simulink model "gm_gmStateSpaceHDL_HalfWaveRectifier_HDL"  (R2020b)
settings: Solver=FixedStepDiscrete  StartTime=0.0  StopTime=5*tin  RelTol=1e-3  AbsTol=1e-3
InitFcn:
  | ts = 1e-6; % local solver sample time
  | tin = 100*ts; % input time period
  | load('/home/ts/Dokumente/ultrazohm_testbench/ultrazohm_test/ultrazohm_sw/ip_cores/simscapeHDL_example_v1_0/sschdl/HalfWaveRectifier_HDL/stateSpaceParameters.mat');
libraries: hdlmdlgenlib x16, dspsigops x10, simulink x7, hdlssclib x3
settings Model: Creator=The MathWorks, Inc.  LastModifiedBy=ts
settings SolverCC: AutoScaleAbsTol=off
settings DataIOCC: SaveOutput=off  SaveTime=off  ReturnWorkspaceOutputs=off
settings OptimizationCC: BlockReduction=off  ConditionallyExecuteInputs=off  DefaultParameterBehavior=Inlined
settings DebuggingCC: AlgebraicLoopMsg=error  InheritedTsInSrcMsg=none  SingleTaskRateTransMsg=error  PregeneratedLibrarySubsystemCodeDiagnostic=none  ArithmeticOperatorsInVariantConditions=warning
settings HardwareCC: ProdBitPerPointer=32  ProdBitPerSizeT=32  ProdBitPerPtrDiffT=32  ProdLargestAtomicFloat=None  ProdIntDivRoundTo=Undefined  ProdEndianess=Unspecified  ProdWordSize=32  ProdHWDeviceType=ASIC/FPGA->ASIC/FPGA  TargetBitPerLong=64  TargetBitPerPointer=64  TargetBitPerSizeT=64  TargetBitPerPtrDiffT=64  TargetLongLongMode=on  TargetIntDivRoundTo=Zero  TargetEndianess=LittleEndian  TargetWordSize=64  TargetHWDeviceType=Custom Processor->MATLAB Host Computer  ProdEqTarget=off
settings SFSimCC: SimUseLocalCustomCode=off  CustomCodeUndefinedFunction=UseInterfaceOnly
settings RTWCC: RTWUseLocalCustomCode=off
settings CodeAppCC: StateflowObjectComments=on
settings SimscapeCC: SimscapeNormalizeSystem=off  SimscapeNominalValues="[{\"value\":\"10\",\"unit\":\"V\"},{\"value\":\"1\",\"unit\":\"A\"},{\"value\":\"10\",\"unit\":\"N*m\"},{\"value\":\"10\",\"unit\":\"bar\"},{\"value\":\"100\",\"unit\":\"kJ/kg\"},{\"value\":\"1\",\"unit\":\"kW\"},{\"value\":\"300\",\"unit\":\"K\"},{\"value\":\"100\",\"unit\":\"cm^3/s\"},{\"value\":\"1\",\"unit\":\"kN\"},{\"value\":\"1\",\"unit\":\"g/cm^3\"},{\"value\":\"1\",\"unit\":\"l\"},{\"value\":\"1\",\"unit\":\"cm^2\"},{\"value\":\"60\",\"unit\":\"Hz\"}]"  SimscapeLogType=all  SimscapeLogDataHistory=10000

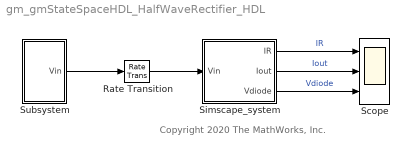
== system gm_gmStateSpaceHDL_HalfWaveRectifier_HDL ==
  note: Copyright 2020 The MathWorks, Inc.
  Rate Transition : RateTransition
  Scope : Scope  NumInputPorts=3
  Simscape_system : Subsystem  TreatAsAtomicUnit=on
  Subsystem : Subsystem
  wires:
  Simscape_system/1(IR) -> Scope/1  "IR"
  Simscape_system/2(Iout) -> Scope/2  "Iout"
  Simscape_system/3(Vdiode) -> Scope/3  "Vdiode"
  Rate Transition/1 -> Simscape_system/1(Vin)
  Subsystem/1(Vin) -> Rate Transition/1

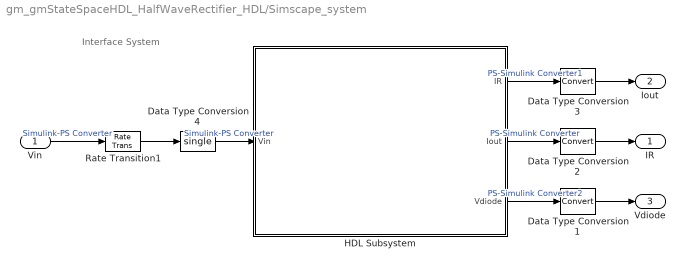
== system gm_gmStateSpaceHDL_HalfWaveRectifier_HDL/Simscape_system ==
  note: Interface System
  Vin : Inport
  Data Type Conversion1 : DataTypeConversion
  Data Type Conversion2 : DataTypeConversion
  Data Type Conversion3 : DataTypeConversion
  Data Type Conversion4 : DataTypeConversion  OutDataTypeStr=single
  HDL Subsystem : Subsystem  TreatAsAtomicUnit=on
  Rate Transition1 : RateTransition  OutPortSampleTime=1e-06
  IR : Outport  VectorParamsAs1DForOutWhenUnconnected=off
  Iout : Outport  Port=2  VectorParamsAs1DForOutWhenUnconnected=off
  Vdiode : Outport  Port=3  VectorParamsAs1DForOutWhenUnconnected=off
  wires:
  Vin/1 -> Rate Transition1/1  "Simulink-PS Converter"
  HDL Subsystem/1(IR) -> Data Type Conversion3/1  "PS-Simulink Converter1"
  HDL Subsystem/2(Iout) -> Data Type Conversion2/1  "PS-Simulink Converter"
  HDL Subsystem/3(Vdiode) -> Data Type Conversion1/1  "PS-Simulink Converter2"
  Data Type Conversion4/1 -> HDL Subsystem/1(Vin)  "Simulink-PS Converter"
  Data Type Conversion1/1 -> Vdiode/1
  Rate Transition1/1 -> Data Type Conversion4/1
  Data Type Conversion3/1 -> Iout/1
  Data Type Conversion2/1 -> IR/1

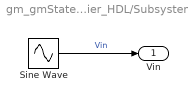
== system gm_gmStateSpaceHDL_HalfWaveRectifier_HDL/Subsystem ==
  Sine Wave : Sin  Amplitude=10  Frequency=2*pi/(tin)  SampleTime=0
  Vin : Outport  VectorParamsAs1DForOutWhenUnconnected=off
  wires:
  Sine Wave/1 -> Vin/1  "Vin"

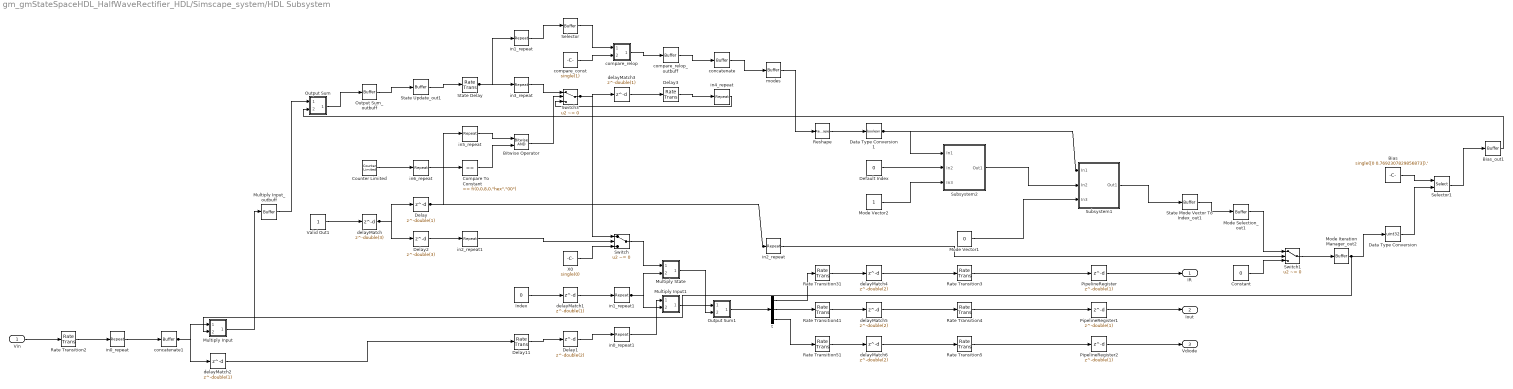
== system gm_gmStateSpaceHDL_HalfWaveRectifier_HDL/Simscape_system/HDL Subsystem ==
  Vin : Inport  OutDataTypeStr=single  PortDimensions=1  SampleTime=1e-06
  Bias : Constant  Value=single([0 0.7692307829856873]).'  OutDataTypeStr=single  SampleTime=5.55555555555556e-09
  Bias_out1 : hdlmdlgenlib/Buffer
      settings: SourceProductBaseCode=SL
  Bitwise Operator : simulink/Logic and Bit Operations/Bitwise Operator  logicop=AND  UseBitMask=off  NumInputPorts=2  BitMask=double(0)  BitMaskRealWorld=Real World Value
  Compare To Constant : simulink/Logic and Bit Operations/Compare To Constant  relop===  const="fi(0,0,8,0,\"hex\",\"00\")"  OutDataTypeStr=boolean
  Constant : Constant  Value=0  OutDataTypeStr=fixdt(0, 1, 0)  SampleTime=5.55555555555556e-09
  Counter Limited : simulink/Sources/Counter Limited  uplimit=double(2)  tsamp=3.33333333333333e-07
  Data Type Conversion : DataTypeConversion  OutDataTypeStr=uint32  SampleTime=5.55555555555556e-09
  Data Type Conversion1 : DataTypeConversion  OutDataTypeStr=boolean  SampleTime=5.55555555555556e-09
  Default Index : Constant  Value=0  OutDataTypeStr=fixdt(0, 1, 0)  SampleTime=5.55555555555556e-09
  Delay : Delay  DelayLength=double(1)  InitialCondition=0  SampleTime=3.33333333333333e-07
  Delay1 : Delay  DelayLength=double(2)  InitialCondition=0  SampleTime=3.33333333333333e-07
  Delay11 : RateTransition  OutPortSampleTimeOpt=Multiple of input port sample time  OutPortSampleTimeMultiple=60
  Delay2 : Delay  DelayLength=double(3)  InitialCondition=0  SampleTime=3.33333333333333e-07
  Delay3 : RateTransition  OutPortSampleTimeOpt=Multiple of input port sample time  OutPortSampleTimeMultiple=60
  Index : Constant  Value=0  OutDataTypeStr=fixdt(0, 1, 0)  SampleTime=3.33333333333333e-07
  Mode Iteration Manager_out2 : hdlmdlgenlib/Buffer
      settings: SourceProductBaseCode=SL
  Mode Selection_out1 : hdlmdlgenlib/Buffer
      settings: SourceProductBaseCode=SL
  Mode Vector1 : Constant  Value=0  OutDataTypeStr=boolean  SampleTime=5.55555555555556e-09
  Mode Vector2 : Constant  OutDataTypeStr=boolean  SampleTime=5.55555555555556e-09
  Multiply Input : Subsystem
      mask Display: disp('NFP\nSparseConstMultiply');
  Multiply Input1 : Subsystem
      mask Display: disp('NFP\nSparseConstMultiply');
  Multiply Input_outbuff : hdlmdlgenlib/Buffer
      settings: SourceProductBaseCode=SL
  Multiply State : Subsystem
      mask Display: disp('NFP\nSparseConstMultiply');
  Output Sum : Subsystem
      mask Display: disp('NFP\nadd');
  Output Sum1 : Subsystem
      mask Display: disp('NFP\nadd');
  Output Sum_outbuff : hdlmdlgenlib/Buffer
      settings: SourceProductBaseCode=SL
  PipelineRegister : Delay  DelayLength=double(1)  InitialCondition=0  SampleTime=1e-06
  PipelineRegister1 : Delay  DelayLength=double(1)  InitialCondition=0  SampleTime=1e-06
  PipelineRegister2 : Delay  DelayLength=double(1)  InitialCondition=0  SampleTime=1e-06
  Rate Transition2 : RateTransition  Integrity=off  Deterministic=off  InitialCondition=double(0)  OutPortSampleTimeOpt=Multiple of input port sample time  OutPortSampleTimeMultiple=1/3
  Rate Transition3 : RateTransition  InitialCondition=double(0)  OutPortSampleTimeOpt=Multiple of input port sample time  OutPortSampleTimeMultiple=3
  Rate Transition31 : RateTransition  OutPortSampleTimeOpt=Multiple of input port sample time  OutPortSampleTimeMultiple=60
  Rate Transition4 : RateTransition  InitialCondition=double(0)  OutPortSampleTimeOpt=Multiple of input port sample time  OutPortSampleTimeMultiple=3
  Rate Transition41 : RateTransition  OutPortSampleTimeOpt=Multiple of input port sample time  OutPortSampleTimeMultiple=60
  Rate Transition5 : RateTransition  InitialCondition=double(0)  OutPortSampleTimeOpt=Multiple of input port sample time  OutPortSampleTimeMultiple=3
  Rate Transition51 : RateTransition  OutPortSampleTimeOpt=Multiple of input port sample time  OutPortSampleTimeMultiple=60
  Reshape : Reshape
  Selector : hdlmdlgenlib/Buffer
      settings: SourceProductBaseCode=SL
  Selector1 : Selector  NumberOfDimensions=2  IndexMode=Zero-based  SampleTime=5.55555555555556e-09  IndexOptions=Select all,Index vector (port)  Indices=double([1 3]),[]  OutputSizes=double(1),[]
  State Delay : RateTransition  OutPortSampleTimeOpt=Multiple of input port sample time  OutPortSampleTimeMultiple=60
  State Mode Vector To Index_out1 : hdlmdlgenlib/Buffer
      settings: SourceProductBaseCode=SL
  State Update_out1 : hdlmdlgenlib/Buffer
      settings: SourceProductBaseCode=SL
  Subsystem1 : Subsystem  mask{Index=fi(0,0,1,0,"hex","0")}
  Subsystem2 : Subsystem  mask{Index=fi(0,0,1,0,"hex","1")}
  Switch : Switch  Criteria=u2 ~= 0  Threshold=double(0)  OutDataTypeStr=single  SampleTime=5.55555555555556e-09
  Switch1 : Switch  Criteria=u2 ~= 0  Threshold=double(0)  OutDataTypeStr=fixdt(0, 1, 0)  SampleTime=5.55555555555556e-09
  Switch3 : Switch  Criteria=u2 ~= 0  Threshold=double(0)  OutDataTypeStr=single  SampleTime=5.55555555555556e-09
  Valid Out1 : Constant  OutDataTypeStr=boolean  SampleTime=3.33333333333333e-07
  X0 : Constant  Value=single(0)  OutDataTypeStr=single  SampleTime=5.55555555555556e-09
  compare_const : Constant  Value=single(1)  OutDataTypeStr=single  SampleTime=5.55555555555556e-09
  compare_relop : Subsystem
      mask Display: disp('NFP\nrelop');
  compare_relop_outbuff : hdlmdlgenlib/Buffer
      settings: SourceProductBaseCode=SL
  concatenate : hdlmdlgenlib/Buffer
      settings: SourceProductBaseCode=SL
  concatenate1 : hdlmdlgenlib/Buffer
      settings: SourceProductBaseCode=SL
  delayMatch : Delay  DelayLength=double(3)  InitialCondition=0  SampleTime=3.33333333333333e-07
  delayMatch1 : Delay  DelayLength=double(1)  InitialCondition=0  SampleTime=3.33333333333333e-07
  delayMatch2 : Delay  DelayLength=double(1)  InitialCondition=0  SampleTime=5.55555555555556e-09
  delayMatch3 : Delay  DelayLength=double(1)  InitialCondition=0  SampleTime=5.55555555555556e-09
  delayMatch4 : Delay  DelayLength=double(2)  InitialCondition=0  SampleTime=3.33333333333333e-07
  delayMatch5 : Delay  DelayLength=double(2)  InitialCondition=0  SampleTime=3.33333333333333e-07
  delayMatch6 : Delay  DelayLength=double(2)  InitialCondition=0  SampleTime=3.33333333333333e-07
  in0_repeat : dspsigops/Repeat  N=double(60)  RateOptions=Allow multirate processing  ic=0  mode=Unused parameter value
  in0_repeat1 : dspsigops/Repeat  N=double(60)  RateOptions=Allow multirate processing  ic=0  mode=Unused parameter value
  in1_repeat : dspsigops/Repeat  N=double(60)  RateOptions=Allow multirate processing  ic=0  mode=Unused parameter value
  in1_repeat1 : dspsigops/Repeat  N=double(60)  RateOptions=Allow multirate processing  ic=0  mode=Unused parameter value
  in2_repeat : dspsigops/Repeat  N=double(60)  RateOptions=Allow multirate processing  ic=0  mode=Unused parameter value
  in2_repeat1 : dspsigops/Repeat  N=double(60)  RateOptions=Allow multirate processing  ic=0  mode=Unused parameter value
  in3_repeat : dspsigops/Repeat  N=double(60)  RateOptions=Allow multirate processing  ic=0  mode=Unused parameter value
  in4_repeat : dspsigops/Repeat  N=double(60)  RateOptions=Allow multirate processing  ic=0  mode=Unused parameter value
  in5_repeat : dspsigops/Repeat  N=double(60)  RateOptions=Allow multirate processing  ic=0  mode=Unused parameter value
  in6_repeat : dspsigops/Repeat  N=double(60)  RateOptions=Allow multirate processing  ic=0  mode=Unused parameter value
  modes : hdlmdlgenlib/Buffer
      settings: SourceProductBaseCode=SL
  t : Demux  Outputs=3
  IR : Outport
  Iout : Outport  Port=2
  Vdiode : Outport  Port=3
  wires:
  Vin/1 -> Rate Transition2/1
  Delay11/1 -> Delay1/1
  Rate Transition2/1 -> in0_repeat/1
  PipelineRegister/1 -> IR/1
  PipelineRegister1/1 -> Iout/1
  PipelineRegister2/1 -> Vdiode/1
  Delay1/1 -> in0_repeat1/1
  delayMatch1/1 -> in1_repeat1/1
  State Delay/1 -> in1_repeat/1, in3_repeat/1
  Counter Limited/1 -> in6_repeat/1
  Delay/1 -> in2_repeat/1, in5_repeat/1
  Delay2/1 -> in2_repeat1/1
  delayMatch/1 -> Delay2/1, Delay/1
  delayMatch4/1 -> Rate Transition3/1
  delayMatch5/1 -> Rate Transition4/1
  delayMatch6/1 -> Rate Transition5/1
  Rate Transition3/1 -> PipelineRegister/1
  Rate Transition4/1 -> PipelineRegister1/1
  Rate Transition5/1 -> PipelineRegister2/1
  Rate Transition31/1 -> delayMatch4/1
  Rate Transition41/1 -> delayMatch5/1
  Rate Transition51/1 -> delayMatch6/1
  Delay3/1 -> in4_repeat/1
  Valid Out1/1 -> delayMatch/1
  Index/1 -> delayMatch1/1
  State Update_out1/1 -> State Delay/1
  delayMatch2/1 -> Delay11/1
  in0_repeat/1 -> concatenate1/1
  in1_repeat/1 -> Selector/1
  in2_repeat/1 -> Switch1/2
  Bias/1 -> Selector1/1
  Data Type Conversion/1 -> Selector1/2
  Selector1/1 -> Bias_out1/1
  Output Sum_outbuff/1 -> State Update_out1/1
  Multiply Input_outbuff/1 -> Output Sum/1(In1)
  Mode Iteration Manager_out2/1 -> Multiply Input/2(In2), Data Type Conversion/1
  Default Index/1 -> Subsystem2/2(In2)
  Mode Vector2/1 -> Subsystem2/3(In3)
  Subsystem2/1(Out1) -> Subsystem1/2(In2)
  Selector/1 -> compare_relop/1(In1)
  compare_const/1 -> compare_relop/2(In2)
  compare_relop_outbuff/1 -> concatenate/1
  concatenate/1 -> modes/1
  modes/1 -> Reshape/1
  Reshape/1 -> Data Type Conversion1/1
  Data Type Conversion1/1 -> Subsystem1/1(In1), Subsystem2/1(In1)
  Mode Vector1/1 -> Subsystem1/3(In3)
  Subsystem1/1(Out1) -> State Mode Vector To Index_out1/1
  State Mode Vector To Index_out1/1 -> Mode Selection_out1/1
  Mode Selection_out1/1 -> Switch1/1
  Constant/1 -> Switch1/3
  Switch1/1 -> Mode Iteration Manager_out2/1
  compare_relop/1(Out1) -> compare_relop_outbuff/1
  Output Sum/1(Out1) -> Output Sum_outbuff/1
  Multiply Input/1(Out1) -> Multiply Input_outbuff/1
  Bias_out1/1 -> Output Sum/2(In2)
  concatenate1/1 -> delayMatch2/1, Multiply Input/1(In1)
  delayMatch3/1 -> Delay3/1
  in0_repeat1/1 -> Multiply Input1/1(In1)
  in1_repeat1/1 -> Multiply State/2(In2), Multiply Input1/2(In2)
  in2_repeat1/1 -> Switch/2
  in3_repeat/1 -> Switch3/1
  in4_repeat/1 -> Switch3/3
  in5_repeat/1 -> Bitwise Operator/1
  in6_repeat/1 -> Compare To Constant/1
  X0/1 -> Switch/3
  Switch/1 -> Multiply State/1(In1)
  Compare To Constant/1 -> Bitwise Operator/2
  Bitwise Operator/1 -> Switch3/2
  t/1 -> Rate Transition31/1
  t/2 -> Rate Transition41/1
  t/3 -> Rate Transition51/1
  Multiply Input1/1(Out1) -> Output Sum1/1(In1)
  Output Sum1/1(Out1) -> t/1
  Multiply State/1(Out1) -> Output Sum1/2(In2)
  Switch3/1 -> delayMatch3/1, Switch/1

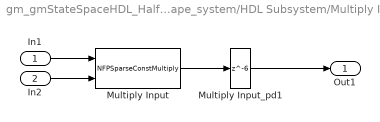
== system gm_gmStateSpaceHDL_HalfWaveRectifier_HDL/Simscape_system/HDL Subsystem/Multiply Input ==
  In1 : Inport
  In2 : Inport  Port=2
  Multiply Input : hdlssclib/NFPSparseConstMultiply  constMatrix="reshape(single([1 0.23076923191547394]).', [1  1  2])"
      settings: SourceProductBaseCode=SL
  Multiply Input_pd1 : Delay  DelayLength=6
  Out1 : Outport
  wires:
  In1/1 -> Multiply Input/1
  In2/1 -> Multiply Input/2
  Multiply Input/1 -> Multiply Input_pd1/1
  Multiply Input_pd1/1 -> Out1/1

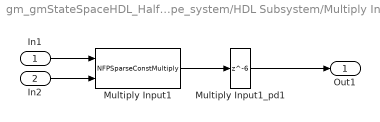
== system gm_gmStateSpaceHDL_HalfWaveRectifier_HDL/Simscape_system/HDL Subsystem/Multiply Input1 ==
  In1 : Inport
  In2 : Inport  Port=2
  Multiply Input1 : hdlssclib/NFPSparseConstMultiply  constMatrix=single([1 1 0]).'
      settings: SourceProductBaseCode=SL
  Multiply Input1_pd1 : Delay  DelayLength=6
  Out1 : Outport
  wires:
  In1/1 -> Multiply Input1/1
  In2/1 -> Multiply Input1/2
  Multiply Input1/1 -> Multiply Input1_pd1/1
  Multiply Input1_pd1/1 -> Out1/1

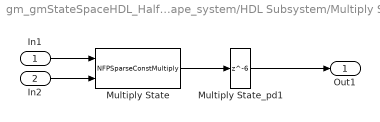
== system gm_gmStateSpaceHDL_HalfWaveRectifier_HDL/Simscape_system/HDL Subsystem/Multiply State ==
  In1 : Inport
  In2 : Inport  Port=2
  Multiply State : hdlssclib/NFPSparseConstMultiply  constMatrix=single([-1 -1 1]).'
      settings: SourceProductBaseCode=SL
  Multiply State_pd1 : Delay  DelayLength=6
  Out1 : Outport
  wires:
  In1/1 -> Multiply State/1
  In2/1 -> Multiply State/2
  Multiply State/1 -> Multiply State_pd1/1
  Multiply State_pd1/1 -> Out1/1

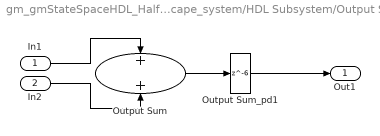
== system gm_gmStateSpaceHDL_HalfWaveRectifier_HDL/Simscape_system/HDL Subsystem/Output Sum ==
  In1 : Inport
  In2 : Inport  Port=2
  Output Sum : Sum  OutDataTypeStr=single  SampleTime=5.55555555555556e-09
  Output Sum_pd1 : Delay  DelayLength=6
  Out1 : Outport
  wires:
  In1/1 -> Output Sum/1
  In2/1 -> Output Sum/2
  Output Sum/1 -> Output Sum_pd1/1
  Output Sum_pd1/1 -> Out1/1

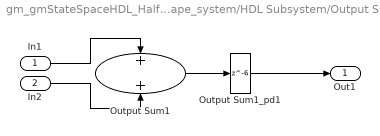
== system gm_gmStateSpaceHDL_HalfWaveRectifier_HDL/Simscape_system/HDL Subsystem/Output Sum1 ==
  In1 : Inport
  In2 : Inport  Port=2
  Output Sum1 : Sum  OutDataTypeStr=single  SampleTime=5.55555555555556e-09
  Output Sum1_pd1 : Delay  DelayLength=6
  Out1 : Outport
  wires:
  In1/1 -> Output Sum1/1
  In2/1 -> Output Sum1/2
  Output Sum1/1 -> Output Sum1_pd1/1
  Output Sum1_pd1/1 -> Out1/1

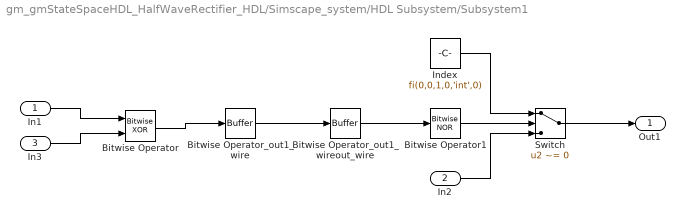
== system gm_gmStateSpaceHDL_HalfWaveRectifier_HDL/Simscape_system/HDL Subsystem/Subsystem1 ==
  In1 : Inport  OutDataTypeStr=boolean  PortDimensions=1  SampleTime=5.55555555555556e-09
  In2 : Inport  Port=2  OutDataTypeStr=fixdt(0, 1, 0)  PortDimensions=1  SampleTime=5.55555555555556e-09
  In3 : Inport  Port=3  OutDataTypeStr=boolean  PortDimensions=1  SampleTime=5.55555555555556e-09
  Bitwise Operator : simulink/Logic and Bit Operations/Bitwise Operator  logicop=XOR  UseBitMask=off  NumInputPorts=2  BitMask=double(0)  BitMaskRealWorld=Real World Value
  Bitwise Operator1 : simulink/Logic and Bit Operations/Bitwise Operator  logicop=NOR  UseBitMask=off  BitMask=double(0)  BitMaskRealWorld=Real World Value
  Bitwise Operator_out1_wire : hdlmdlgenlib/Buffer
      settings: SourceProductBaseCode=SL
  Bitwise Operator_out1_wireout_wire : hdlmdlgenlib/Buffer
      settings: SourceProductBaseCode=SL
  Index : Constant  Value=fi(0,0,1,0,'int',0)  OutDataTypeStr=fixdt(0, 1, 0)  SampleTime=5.55555555555556e-09
  Switch : Switch  Criteria=u2 ~= 0  Threshold=double(0)  OutDataTypeStr=fixdt(0, 1, 0)  SampleTime=5.55555555555556e-09
  Out1 : Outport  VectorParamsAs1DForOutWhenUnconnected=off
  wires:
  Bitwise Operator/1 -> Bitwise Operator_out1_wire/1
  Bitwise Operator1/1 -> Switch/2
  Bitwise Operator_out1_wireout_wire/1 -> Bitwise Operator1/1
  Index/1 -> Switch/1
  Switch/1 -> Out1/1
  Bitwise Operator_out1_wire/1 -> Bitwise Operator_out1_wireout_wire/1
  In1/1 -> Bitwise Operator/1
  In2/1 -> Switch/3
  In3/1 -> Bitwise Operator/2

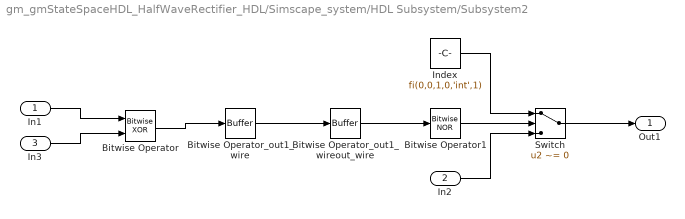
== system gm_gmStateSpaceHDL_HalfWaveRectifier_HDL/Simscape_system/HDL Subsystem/Subsystem2 ==
  In1 : Inport  OutDataTypeStr=boolean  PortDimensions=1  SampleTime=5.55555555555556e-09
  In2 : Inport  Port=2  OutDataTypeStr=fixdt(0, 1, 0)  PortDimensions=1  SampleTime=5.55555555555556e-09
  In3 : Inport  Port=3  OutDataTypeStr=boolean  PortDimensions=1  SampleTime=5.55555555555556e-09
  Bitwise Operator : simulink/Logic and Bit Operations/Bitwise Operator  logicop=XOR  UseBitMask=off  NumInputPorts=2  BitMask=double(0)  BitMaskRealWorld=Real World Value
  Bitwise Operator1 : simulink/Logic and Bit Operations/Bitwise Operator  logicop=NOR  UseBitMask=off  BitMask=double(0)  BitMaskRealWorld=Real World Value
  Bitwise Operator_out1_wire : hdlmdlgenlib/Buffer
      settings: SourceProductBaseCode=SL
  Bitwise Operator_out1_wireout_wire : hdlmdlgenlib/Buffer
      settings: SourceProductBaseCode=SL
  Index : Constant  Value=fi(0,0,1,0,'int',1)  OutDataTypeStr=fixdt(0, 1, 0)  SampleTime=5.55555555555556e-09
  Switch : Switch  Criteria=u2 ~= 0  Threshold=double(0)  OutDataTypeStr=fixdt(0, 1, 0)  SampleTime=5.55555555555556e-09
  Out1 : Outport  VectorParamsAs1DForOutWhenUnconnected=off
  wires:
  Bitwise Operator/1 -> Bitwise Operator_out1_wire/1
  Bitwise Operator1/1 -> Switch/2
  Bitwise Operator_out1_wireout_wire/1 -> Bitwise Operator1/1
  Index/1 -> Switch/1
  Switch/1 -> Out1/1
  Bitwise Operator_out1_wire/1 -> Bitwise Operator_out1_wireout_wire/1
  In1/1 -> Bitwise Operator/1
  In2/1 -> Switch/3
  In3/1 -> Bitwise Operator/2

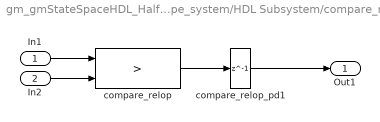
== system gm_gmStateSpaceHDL_HalfWaveRectifier_HDL/Simscape_system/HDL Subsystem/compare_relop ==
  In1 : Inport
  In2 : Inport  Port=2
  compare_relop : RelationalOperator  Operator=>  OutDataTypeStr=boolean  SampleTime=5.55555555555556e-09  RndMeth=Nearest  InputSameDT=on
  compare_relop_pd1 : Delay  DelayLength=1
  Out1 : Outport
  wires:
  In1/1 -> compare_relop/1
  In2/1 -> compare_relop/2
  compare_relop/1 -> compare_relop_pd1/1
  compare_relop_pd1/1 -> Out1/1
